simulink model "disperazione"  (R2022a)
settings: Solver=ode4  StartTime=0.0  StopTime=info.Tsim  FixedStep=0.1  RelTol=1e-15
values from neighbouring files (symbols this model uses):
  condDiscMat = BuildCondendsedMPCmatrices(discreteMat,r,q,F,f,PH)    [MAIN_MIMO.m]    (also in backupMain.m; test.m)
  discreteModel = c2d(continuousModel, info.Ts)    [MAIN_MIMO.m]    (also in backupMain.m; nonLinearPatient_main.m; test.m)
  PH = 100    [MAIN_MIMO.m]    (also in backupMain.m = 200; nonLinearPatient_main.m = 200; test.m = 200)
  R_KF = 0.001*eye(2)    [MAIN_MIMO.m]    (also in backupMain.m; nonLinearPatient_main.m; test.m)
undefined symbols (not defined in the file or in its folder): Discrete, info, myMPC_dist, op, Time
libraries: ctrlSharedLib x1
settings Model: Creator=cionescu  LastModifiedBy=user
settings SolverCC: AlgebraicLoopSolver=TrustRegion
settings DataIOCC: SaveState=on  ReturnWorkspaceOutputs=off
settings DebuggingCC: UnconnectedInputMsg=warning  UnconnectedOutputMsg=warning  UnconnectedLineMsg=warning  SFMachineParentedDataDiag=warning  ArithmeticOperatorsInVariantConditions=warning
settings SFSimCC: SimUseLocalCustomCode=off  CustomCodeUndefinedFunction=UseInterfaceOnly
settings RTWCC: RTWUseLocalCustomCode=off  DLArmComputeVersion=19.05
settings CodeAppCC: StateflowObjectComments=on

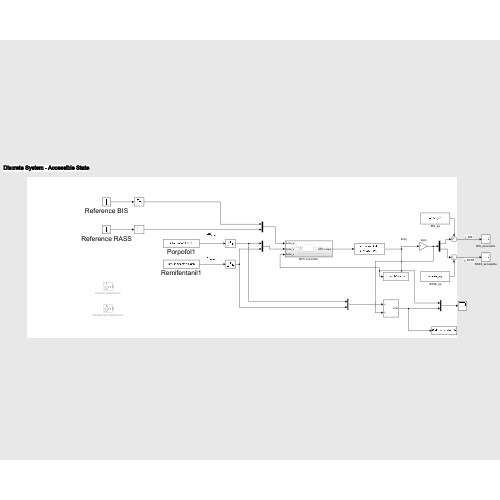
[thumbnail: Simulink's stored preview of the top-level diagram]
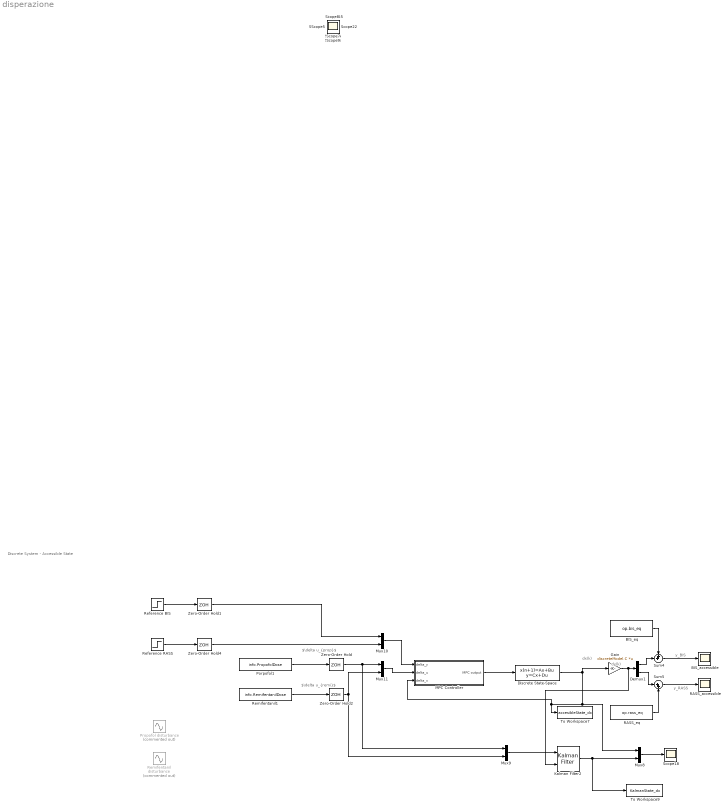
== system disperazione ==
  note: $\delta u_{remi}$
  note: dx(k)
  note: y_RASS
  note: Discrete System - Accessible State
  note: dy(k)
  note: y_BIS
  note: $\delta u_{prop}$
  BIS_accessible : Scope
  BIS_eq : Constant  Value=op.bis_eq
  Demux1 : Demux  Outputs=2
  Discrete State-Space : DiscreteStateSpace  A=discreteModel.A  B=discreteModel.B  C=eye(size(discreteModel.A))  D=zeros(size(discreteModel.A,1),size(discreteModel.B,2))  InitialCondition=[0,0,0,-0.5584,-2,0,0,0,0,0]'  SampleTime=info.Ts
  Gain : Gain  Gain=discreteModel.C  Multiplication=Matrix(K*u)
  Kalman Filter2 : ctrlSharedLib/Kalman Filter  TimeDomain=Discrete-Time  UseCurrentEstimator=on  ModelSource=LTI State-Space Variable  ModelSourceVariable=discreteModel  A=0.95  B=1  C=1  D=0  NumberOfStates=1  NumberOfInputs=1  NumberOfOutputs=1  InitialEstimateSource=Dialog  X0=[0,0,0,-0.5584,-2,0,0,0,0,0]'  P0=10  UseK=off  UseGH=off  NumberOfProcessNoiseInputs=1  G=1  TimeInvariantG=on  H=0  TimeInvariantH=on  Q=Q_KF  TimeInvariantQ=on  R=R_KF  TimeInvariantR=on  N=0  TimeInvariantN=on  AddInputPort=on  AddEnablePort=off  OutputEstimatedY=off  OutputP=off  Ts=-1
  MPC Controller : Subsystem
  Mux{8..11} (4 alike) : Mux  Inputs=2
  Porpofol1 : Constant  Value=info.PropofolDose  SampleTime=info.Ts
  Propofol disturbance : Sin  Commented=on  Amplitude=0.3*op.propofol_eq  Frequency=1/500  SampleTime=info.Ts
  RASS_accessible : Scope
  RASS_eq : Constant  Value=op.rass_eq
  Reference BIS : Step  Time=info.T_induction  Before=50  After=0  SampleTime=info.Ts
  Reference RASS : Step  Time=info.T_induction  Before=4  After=0  SampleTime=info.Ts
  Remifentanil disturbance : Sin  Commented=on  Amplitude=0.3*op.remifentanil_eq  Frequency=1/700  SampleTime=info.Ts
  Remifentanil1 : Constant  Value=info.RemifentanilDose  SampleTime=info.Ts
  Scope{,2,5,7..16,18} (14 alike) : Scope
  Sum4 : Sum  Inputs=++|
  Sum5 : Sum  Inputs=|++
  To Workspace7 : ToWorkspace  VariableName=accesibleState_dx  SaveFormat=Structure With Time  SampleTime=-1
  To Workspace9 : ToWorkspace  VariableName=KalmanState_dx  SaveFormat=Structure With Time  SampleTime=-1
  Zero-Order Hold{,1..2,4} (4 alike) : ZeroOrderHold  SampleTime=info.Ts
  wires:
  BIS_eq/1 -> Sum4/1
  Demux1/2 -> Sum5/1
  RASS_eq/1 -> Sum5/2
  Demux1/1 -> Sum4/2
  Gain/1 -> Kalman Filter2/2, Demux1/1
  Sum5/1 -> RASS_accessible/1
  Sum4/1 -> BIS_accessible/1
  Discrete State-Space/1 -> Gain/1, MPC Controller/3(delta_x), To Workspace7/1, Mux8/1
  Mux8/1 -> Scope18/1
  Kalman Filter2/1 -> To Workspace9/1, Mux8/2
  Mux9/1 -> Kalman Filter2/1
  Porpofol1/1 -> Zero-Order Hold/1
  Remifentanil1/1 -> Zero-Order Hold2/1
  Reference BIS/1 -> Zero-Order Hold1/1
  Reference RASS/1 -> Zero-Order Hold4/1
  Zero-Order Hold1/1 -> Mux10/1
  Zero-Order Hold4/1 -> Mux10/2
  Mux10/1 -> MPC Controller/1(delta_y)
  Mux11/1 -> MPC Controller/2(delta_u)
  MPC Controller/1(MPC output) -> Discrete State-Space/1
  Zero-Order Hold/1 -> Mux9/1, Mux11/1
  Zero-Order Hold2/1 -> Mux9/2, Mux11/2

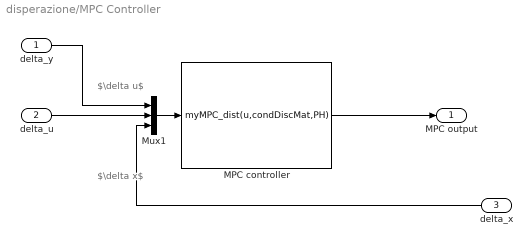
== system disperazione/MPC Controller ==
  note: $\delta x$
  note: $\delta u$
  delta_y : Inport
  delta_u : Inport  Port=2
  delta_x : Inport  Port=3
  MPC controller : MATLABFcn  MATLABFcn=myMPC_dist(u,condDiscMat,PH)  OutputDimensions=2
  Mux1 : Mux  Inputs=3
  MPC output : Outport
  wires:
  delta_x/1 -> Mux1/3
  Mux1/1 -> MPC controller/1
  MPC controller/1 -> MPC output/1
  delta_u/1 -> Mux1/2
  delta_y/1 -> Mux1/1
